simulink model "Feedforward_ROS"  (R2022b)
settings: Solver=FixedStepAuto  StartTime=0.0  StopTime=Inf  FixedStep=0.02  MaxStep=0.1  RelTol=1e-3
undefined symbols (not defined in the file): unicycle, X, Y
libraries: robotlib x3, simulink_extras x2
settings Model: Creator=hp 2021  LastModifiedBy=mustacchim
settings OptimizationCC: EnhancedBackFolding=on  PassReuseOutputArgsAs=Individual arguments  ZeroExternalMemoryAtStartup=off  ZeroInternalMemoryAtStartup=off  MaxStackSize=64  OptimizeBlockOrder=speed  DifferentSizesBufferReuse=on  OptimizationCustomize=off  EfficientTunableParamExpr=on
settings DebuggingCC: ParameterTunabilityLossMsg=error
settings HardwareCC: ProdBitPerPointer=32  ProdBitPerSizeT=32  ProdBitPerPtrDiffT=32  ProdLargestAtomicFloat=None  ProdIntDivRoundTo=Undefined  ProdEndianess=Unspecified  ProdWordSize=32  ProdHWDeviceType=Generic->Unspecified (assume 32-bit Generic)  UseEmbeddedCoderFeatures=off
settings ModelReferenceCC: EnableRefExpFcnMdlSchedulingChecks=on
settings SFSimCC: MATLABDynamicMemAlloc=off
settings RTWCC: Description=Embedded Coder  SystemTargetFile=ert.tlc  HardwareBoard=Robot Operating System (ROS)  TLCOptions="-aInlineSetEventsForThisBaseRateFcn=TLC_FALSE -aSuppressMultiTaskScheduler=TLC_FALSE  -aRateBasedStepFcn=0"  TemplateMakefile=ert_default_tmf  Toolchain=Catkin  TargetLang=C++
settings CodeAppCC: ForceParamTrailComments=on  IgnoreCustomStorageClasses=off  OperatorAnnotations=on  SimulinkDataObjDesc=on  SFDataObjDesc=on  InsertBlockDesc=on
settings ERTTargetCC: SupportNonInlinedSFcns=on

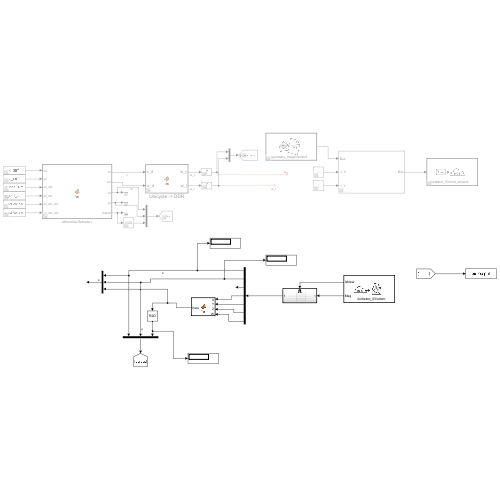
[thumbnail: Simulink's stored preview of the top-level diagram]
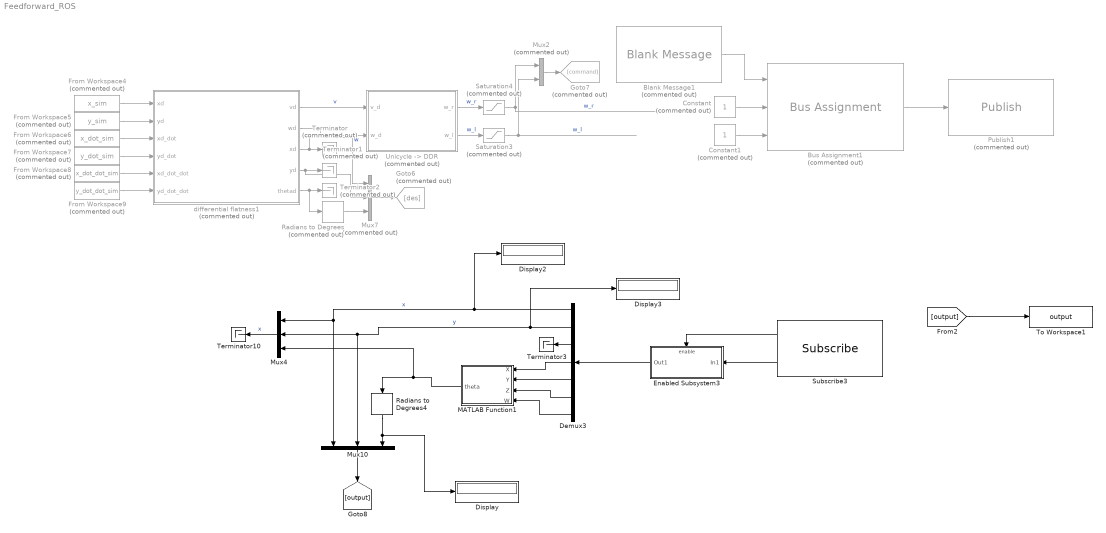
== system Feedforward_ROS ==
  Blank Message1 : robotlib/Blank Message  Commented=on  messageClass=Message  entityType=geometry_msgs/Vector3  messageType=geometry_msgs/Vector3  SampleTime=0.02  legacyBusStruct=off
      settings: LibrarySourceBlock=roslib/ROS/Blank Message
  Bus Assignment1 : BusAssignment  Commented=on  AssignedSignals=X,Y
  Constant : Constant  Commented=on
  Constant1 : Constant  Commented=on
  Demux3 : Demux  Outputs=7
  Display : Display
  Display2 : Display
  Display3 : Display
  Enabled Subsystem3 : Subsystem  TreatAsAtomicUnit=on
  From Workspace4 : FromWorkspace  Commented=on  VariableName=x_sim
  From Workspace5 : FromWorkspace  Commented=on  VariableName=y_sim
  From Workspace6 : FromWorkspace  Commented=on  VariableName=x_dot_sim
  From Workspace7 : FromWorkspace  Commented=on  VariableName=y_dot_sim
  From Workspace8 : FromWorkspace  Commented=on  VariableName=x_dot_dot_sim
  From Workspace9 : FromWorkspace  Commented=on  VariableName=y_dot_dot_sim
  Goto6 : Goto  Commented=on  GotoTag=des
  Goto7 : Goto  Commented=on  GotoTag=command
  MATLAB Function1 : MATLAB Function  TreatAsAtomicUnit=on
  Mux10 : Mux  Inputs=3
  Mux2 : Mux  Commented=on  Inputs=2
  Mux4 : Mux  Inputs=3
  Mux7 : Mux  Commented=on  Inputs=3
  Publish1 : robotlib/Publish  Commented=on  topicSource=Select from ROS network  topic=/turtlebot_03/cmd_wheels  messageType=geometry_msgs/Vector3  legacyBusStruct=off  messageQueueLength=1
      settings: LibrarySourceBlock=roslib/ROS/Publish
  Radians to Degrees : simulink_extras/Transformations/Radians to Degrees  Commented=on
  Radians to Degrees4 : simulink_extras/Transformations/Radians to Degrees
  Saturation3 : Saturate  Commented=on  UpperLimit=unicycle.omegaWheelMax  LowerLimit=unicycle.omegaWheelMin
  Saturation4 : Saturate  Commented=on  UpperLimit=unicycle.omegaWheelMax  LowerLimit=unicycle.omegaWheelMin
  Subscribe3 : robotlib/Subscribe  topicSource=Select from ROS network  topic=/turtlebot_03/odom  messageType=nav_msgs/Odometry  SampleTime=0.02  legacyBusStruct=off  messageQueueLength=1
      settings: LibrarySourceBlock=roslib/ROS/Subscribe
  Terminator : Terminator  Commented=on
  Terminator1 : Terminator  Commented=on
  Terminator10 : Terminator
  Terminator2 : Terminator  Commented=on
  Terminator3 : Terminator
  To Workspace1 : ToWorkspace  VariableName=output  SaveFormat=Structure With Time  SampleTime=-1
  "Unicycle -> DDR" : MATLAB Function  Commented=on  TreatAsAtomicUnit=on
  differential flatness1 : MATLAB Function  Commented=on  TreatAsAtomicUnit=on
  wires:
  From Workspace8/1 -> differential flatness1/5(xd_dot_dot)
  differential flatness1/5(thetad) -> Radians to Degrees/1, Terminator2/1
  From Workspace9/1 -> differential flatness1/6(yd_dot_dot)
  From Workspace7/1 -> differential flatness1/4(yd_dot)
  From Workspace6/1 -> differential flatness1/3(xd_dot)
  [output] -> To Workspace1/1
  From Workspace4/1 -> differential flatness1/1("xd ")
  From Workspace5/1 -> differential flatness1/2("yd ")
  Blank Message1/1 -> Bus Assignment1/1
  differential flatness1/1(vd) -> "Unicycle -> DDR"/1(v_d)  "v"
  "Unicycle -> DDR"/2(w_l) -> Saturation3/1  "w_l"
  Mux2/1 -> Goto7/1
  Bus Assignment1/1 -> Publish1/1
  Saturation3/1 -> Mux2/2  "w_l"
  Saturation4/1 -> Mux2/1  "w_r"
  "Unicycle -> DDR"/1(w_r) -> Saturation4/1  "w_r"
  differential flatness1/2(wd) -> "Unicycle -> DDR"/2(w_d)  "w"
  Mux4/1 -> Terminator10/1  "x"
  Mux10/1 -> [output]
  Demux3/1 -> Display2/1, Mux4/1, Mux10/1  "x"
  Subscribe3/2 -> Enabled Subsystem3/1(In1)
  Radians to Degrees4/1 -> Display/1, Mux10/3
  Subscribe3/1 -> Enabled Subsystem3/Enable
  Demux3/2 -> Display3/1, Mux10/2, Mux4/2  "y"
  Enabled Subsystem3/1(Out1) -> Demux3/1
  Mux7/1 -> Goto6/1
  differential flatness1/4(yd) -> Mux7/2, Terminator1/1
  differential flatness1/3(xd) -> Mux7/1, Terminator/1
  Radians to Degrees/1 -> Mux7/3
  Demux3/7 -> MATLAB Function1/4(W)
  Demux3/3 -> Terminator3/1
  MATLAB Function1/1(theta) -> Mux4/3, Radians to Degrees4/1
  Demux3/4 -> MATLAB Function1/1(X)
  Demux3/6 -> MATLAB Function1/3(Z)
  Demux3/5 -> MATLAB Function1/2(Y)
  Constant/1 -> Bus Assignment1/2
  Constant1/1 -> Bus Assignment1/3

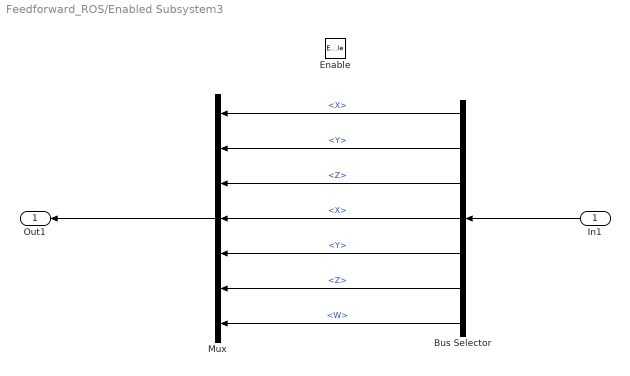
== system Feedforward_ROS/Enabled Subsystem3 ==
  In1 : Inport
  Enable : EnablePort
  Bus Selector : BusSelector  OutputSignals=Pose.Pose.Position.X,Pose.Pose.Position.Y,Pose.Pose.Position.Z,Pose.Pose.Orientation.X,Pose.Pose.Orientation.Y,Pose.Pose.Orientation.Z,Pose.Pose.Orientation.W
  Mux : Mux  Inputs=7
  Out1 : Outport
  wires:
  Mux/1 -> Out1/1
  Bus Selector/1 -> Mux/1  "<X>"
  Bus Selector/2 -> Mux/2  "<Y>"
  In1/1 -> Bus Selector/1
  Bus Selector/3 -> Mux/3  "<Z>"
  Bus Selector/4 -> Mux/4  "<X>"
  Bus Selector/5 -> Mux/5  "<Y>"
  Bus Selector/6 -> Mux/6  "<Z>"
  Bus Selector/7 -> Mux/7  "<W>"

== matlab function Feedforward_ROS/MATLAB Function1 ==
  data: X input; Y input; Z input; theta output; W input
function theta = fcn(X, Y, Z, W)

    q_x = X;
    q_y = Y;
    q_z = Z;
    q_w = W;
    
    q = cat(2,q_w,q_x,q_y,q_z); 
    eulZYX = quat2eul(q,'ZYX');
    theta = eulZYX(1);
    
end

== matlab function Feedforward_ROS/differential flatness1 ==
  data: xd input; vd output; yd input; xd_dot input; yd_dot input; xd_dot_dot input; yd_dot_dot input; wd output; xd output; yd output; thetad output
function [vd, wd, xd, yd, thetad] = fcn(xd, yd, xd_dot, yd_dot, xd_dot_dot, yd_dot_dot)
    
    vd = sqrt(xd_dot.^2 + yd_dot.^2);
    wd = (xd_dot.*yd_dot_dot - xd_dot_dot.*yd_dot) / (xd_dot.^2 + yd_dot.^2);
    % thetad = atan2(yd_dot, xd_dot);
    thetad = mod(atan2(yd_dot,xd_dot), 2*pi);

    xd = xd;
    yd = yd;

end

== matlab function Feedforward_ROS/Unicycle -> DDR ==
  data: v_d input; w_r output; w_d input; w_l output
function [w_r, w_l] = fcn(v_d, w_d)

    %#codegen
    coder.extrinsic('evalin')
    d = 0;                  % Needed in order to set variable class correctly
    r = 0;                  % Needed in order to set variable class correctly
    d = evalin('base','unicycle.d'); % Read value from workspace
    r = evalin('base','unicycle.r'); % Read value from workspace

    w_r = ((2 * v_d) + (w_d * d)) / (2 * r);
    w_l = ((2 * v_d) - (w_d * d)) / (2 * r);

end
